simulink model "Lab_4_simple_corr_completed"  (R2016b)
settings: Solver=FixedStepDiscrete  StartTime=0.0  StopTime=1  RelTol=1e-3
PreLoadFcn:
  | load dspafxr;
libraries: dspsrcs4 x3, dspstat3 x2
settings Model: Creator=sv7  LastModifiedBy=Cemal
settings SolverCC: PositivePriorityOrder=on
settings DataIOCC: SaveFormat=Array  SignalLoggingSaveFormat=ModelDataLogs  SaveOutput=off  SaveTime=off
settings OptimizationCC: DefaultParameterBehavior=Inlined  InlineInvariantSignals=on  ExpressionDepthLimit=2147483647  InitFltsAndDblsToZero=on  LifeSpan=1
settings DebuggingCC: SaveWithParameterizedLinksMsg=none  UnderspecifiedInitializationDetection=Classic  MergeDetectMultiDrivingBlocksExec=none  SignalResolutionControl=TryResolveAllWithWarning  SolverPrmCheckMsg=warning  MultiTaskDSMMsg=warning  MultiTaskCondExecSysMsg=none  FcnCallInpInsideContextMsg=warning  StateNameClashWarn=warning  SFUnexpectedBacktrackingDiag=warning  SFNoUnconditionalDefaultTransitionDiag=warning  SFExecutionAtInitializationDiag=none
settings HardwareCC: ProdBitPerLong=40  ProdBitPerPointer=32  ProdBitPerSizeT=32  ProdBitPerPtrDiffT=32  ProdLargestAtomicInteger=Integer  ProdLargestAtomicFloat=None  ProdWordSize=32  ProdHWDeviceType=Texas Instruments->C6000  TargetBitPerLong=40  TargetLargestAtomicInteger=Integer  TargetIntDivRoundTo=Zero  TargetEndianess=LittleEndian  TargetHWDeviceType=TI C6000
settings ModelReferenceCC: PropagateSignalLabelsOutOfModel=off
settings RTWCC: SystemTargetFile=idelink_ert.tlc  GenerateMakefile=off  TemplateMakefile=none  Description=IDE Link ERT
settings CodeAppCC: IgnoreCustomStorageClasses=off
settings ConfigComp: CovMetricSettings=dw  CovHtmlReporting=on  CovSaveCumulativeToWorkspaceVar=on  CovSaveSingleToWorkspaceVar=on  CovExternalEMLEnable=off
settings TargetHardwareResources: Description=Target Hardware Resources Component

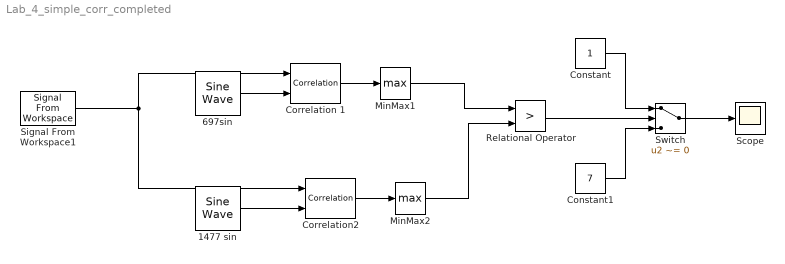
== system Lab_4_simple_corr_completed ==
  1477 sin : dspsrcs4/Sine Wave  Amplitude=1  Frequency=1477  Phase=0  SampleMode=Discrete  OutComplex=Real  CompMethod=Trigonometric fcn  TableSize=Speed  SampleTime=1/8000  SamplesPerFrame=40  ResetState=Restart at time zero  OutputFrames=on  dataType=double  wordLen=16  udDataType=sfix(16)  fracBitsMode=Best precision  numFracBits=15  OutDataTypeStr=double  LastOutDataTypeStr=double
  697sin : dspsrcs4/Sine Wave  Amplitude=1  Frequency=697  Phase=0  SampleMode=Discrete  OutComplex=Real  CompMethod=Trigonometric fcn  TableSize=Speed  SampleTime=1/8000  SamplesPerFrame=40  ResetState=Restart at time zero  OutputFrames=on  dataType=double  wordLen=16  udDataType=sfix(16)  fracBitsMode=Best precision  numFracBits=15  OutDataTypeStr=double  LastOutDataTypeStr=double
  Constant : Constant
  Constant1 : Constant  Value=7
  Correlation 1 : dspstat3/Correlation  domain=Time  roundingMode=Floor  overflowMode=off  outputDataTypeStr=Inherit: Same as accumulator  outputMin=[]  outputMax=[]  outputLastDataTypeStr=Inherit: Same as accumulator
  Correlation2 : dspstat3/Correlation  domain=Time  roundingMode=Floor  overflowMode=off  outputDataTypeStr=Inherit: Same as accumulator  outputMin=[]  outputMax=[]  outputLastDataTypeStr=Inherit: Same as accumulator
  MinMax1 : MinMax  Function=max
  MinMax2 : MinMax  Function=max
  Relational Operator : RelationalOperator  Operator=>  OutDataTypeStr=boolean  RndMeth=Nearest
  Scope : Scope
  Signal From Workspace1 : dspsrcs4/Signal From Workspace  X=SinWave  Ts=1/8000  nsamps=40  OutputAfterFinalValue=Cyclic repetition  ignoreOrWarnInputAndFrameLengths=off  OutputFrames=on
  Switch : Switch  Criteria=u2 ~= 0
  wires:
  Switch/1 -> Scope/1
  Relational Operator/1 -> Switch/2
  Constant1/1 -> Switch/3
  Constant/1 -> Switch/1
  Signal From Workspace1/1 -> Correlation2/1, Correlation 1/1
  1477 sin/1 -> Correlation2/2
  697sin/1 -> Correlation 1/2
  Correlation2/1 -> MinMax2/1
  Correlation 1/1 -> MinMax1/1
  MinMax2/1 -> Relational Operator/2
  MinMax1/1 -> Relational Operator/1
